simulink model "AirRefueling_Platform"  (R2022a)
settings: Solver=ode4  StartTime=0.0  StopTime=inf  FixedStep=0.01  RelTol=1e-5  AbsTol=1e-4  EnableMultiTasking=on
InitFcn:
  | F16_Init
values from neighbouring files (symbols this model uses):
  airSpeed = 393.72    [F16_Init.m]
  altitude = 9843    [F16_Init.m]
  d_f_rc = [3.75;0;-1.75]    [F16_Init.m]
  d_pr_cam = d_pr_rc - d_cam_rc    [F16_Init.m]
  d_pr_rc = [7.6;0.50;-2.44]    [F16_Init.m]
  p0_rc = [-250;-119;0]    [F16_Init.m]
  visual_err = [0.07;0.04;-1.21]    [F16_Init.m]
undefined symbols (not defined in the file or in its folder): Cdr_, dtheta10, dtheta20, F, height, k_reel, kd, l0, l1, l_density, Light, m0, Mdr, MIL, N, Rdr, Rl, STD, T_reel_initial, theta10, theta20, vt0
libraries: etargetslib x10, dspnetwork x10, simulink x2, aerolibconvert2 x2, aerolibwind2 x2, aerolibatmos2 x1, aerolibanimutils x1, slrealtimeiplib x1
(part 2 of 2)

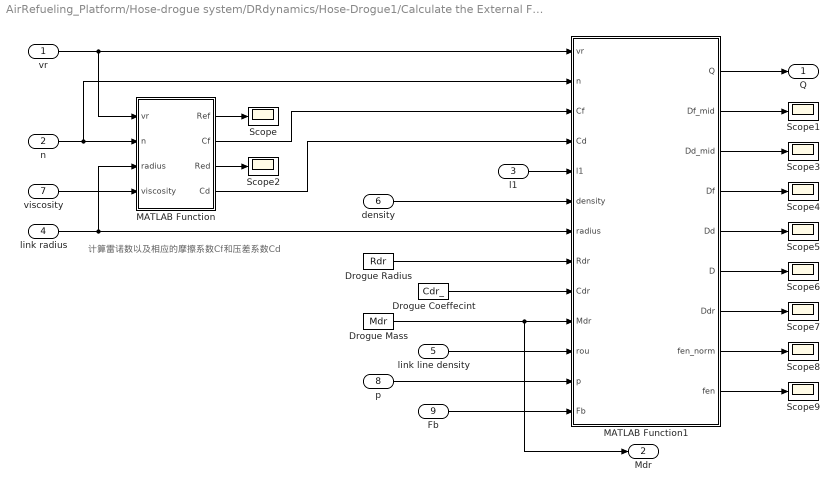
== system AirRefueling_Platform/Hose-drogue system/DRdynamics/Hose-Drogue1/Calculate the External Force of the Links ==
  note: 计算雷诺数以及相应的摩擦系数Cf和压差系数Cd
  vr : Inport
  n : Inport  Port=2
  l1 : Inport  Port=3
  link radius : Inport  Port=4
  link line density : Inport  Port=5
  density : Inport  Port=6
  viscosity : Inport  Port=7
  p : Inport  Port=8
  Fb : Inport  Port=9
  Drogue Coeffecint : Constant  Value=Cdr_
  Drogue Mass : Constant  Value=Mdr
  Drogue Radius : Constant  Value=Rdr
  MATLAB Function : MATLAB Function  TreatAsAtomicUnit=on
  MATLAB Function1 : MATLAB Function  TreatAsAtomicUnit=on
  Scope{,1..9} (10 alike) : Scope
  Q : Outport
  Mdr : Outport  Port=2
  wires:
  MATLAB Function/1(Ref) -> Scope/1
  MATLAB Function/3(Red) -> Scope2/1
  MATLAB Function1/1(Q) -> Q/1
  vr/1 -> MATLAB Function/1(vr), MATLAB Function1/1(vr)
  n/1 -> MATLAB Function1/2(n), MATLAB Function/2(n)
  link radius/1 -> MATLAB Function/3(radius), MATLAB Function1/7(radius)
  viscosity/1 -> MATLAB Function/4(viscosity)
  density/1 -> MATLAB Function1/6(density)
  Drogue Radius/1 -> MATLAB Function1/8(Rdr)
  Drogue Coeffecint/1 -> MATLAB Function1/9(Cdr)
  Drogue Mass/1 -> Mdr/1, MATLAB Function1/10(Mdr)
  link line density/1 -> MATLAB Function1/11(rou)
  MATLAB Function1/2(Df_mid) -> Scope1/1
  MATLAB Function1/3(Dd_mid) -> Scope3/1
  MATLAB Function1/4(Df) -> Scope4/1
  MATLAB Function1/5(Dd) -> Scope5/1
  MATLAB Function1/6(D) -> Scope6/1
  MATLAB Function1/7(Ddr) -> Scope7/1
  MATLAB Function/2(Cf) -> MATLAB Function1/3(Cf)
  MATLAB Function/4(Cd) -> MATLAB Function1/4(Cd)
  p/1 -> MATLAB Function1/12(p)
  l1/1 -> MATLAB Function1/5(l1)
  Fb/1 -> MATLAB Function1/13(Fb)
  MATLAB Function1/8(fen_norm) -> Scope8/1
  MATLAB Function1/9(fen) -> Scope9/1

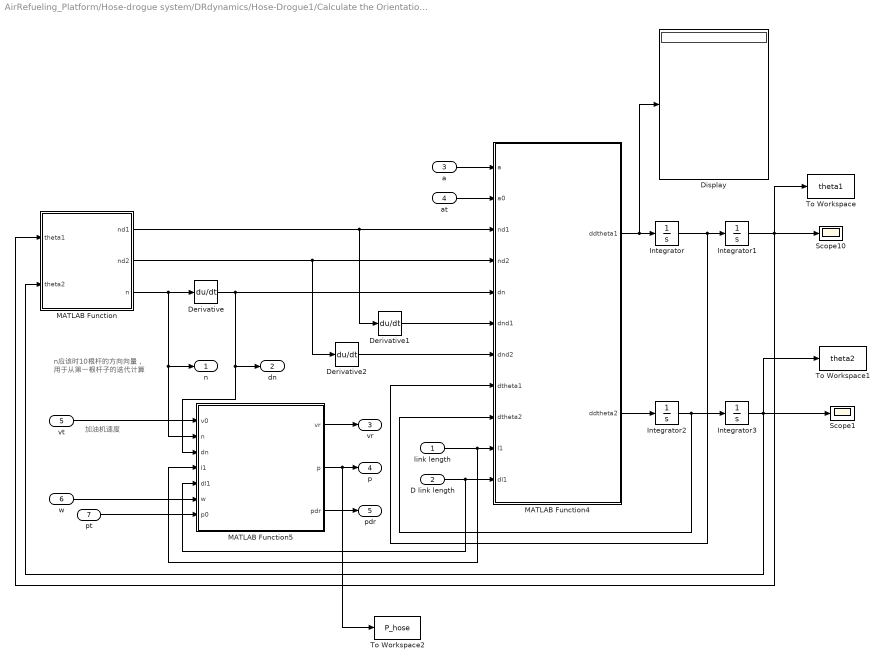
== system AirRefueling_Platform/Hose-drogue system/DRdynamics/Hose-Drogue1/Calculate the Orientation of the Links1 ==
  note: n应该时10根杆的方向向量，
      | 用于从第一根杆子的迭代计算
  note: 加油机速度
  link length : Inport
  D link length : Inport  Port=2
  a : Inport  Port=3
  at : Inport  Port=4
  vt : Inport  Port=5
  w : Inport  Port=6
  pt : Inport  Port=7
  Derivative : Derivative
  Derivative1 : Derivative
  Derivative2 : Derivative
  Display : Display
  Integrator : Integrator  InitialCondition=dtheta10
  Integrator1 : Integrator  InitialCondition=theta10
  Integrator2 : Integrator  InitialCondition=dtheta20
  Integrator3 : Integrator  InitialCondition=theta20
  MATLAB Function : MATLAB Function  TreatAsAtomicUnit=on
  MATLAB Function4 : MATLAB Function  TreatAsAtomicUnit=on
  MATLAB Function5 : MATLAB Function  TreatAsAtomicUnit=on
  Scope1 : Scope
  Scope10 : Scope
  To Workspace : ToWorkspace  VariableName=theta1  SampleTime=-1
      settings: Save2DSignal=2-D array (concatenate along first dimension)
  To Workspace1 : ToWorkspace  VariableName=theta2  SampleTime=-1
      settings: Save2DSignal=2-D array (concatenate along first dimension)
  To Workspace2 : ToWorkspace  VariableName=P_hose  SampleTime=-1
  n : Outport
  dn : Outport  Port=2
  vr : Outport  Port=3
  p : Outport  Port=4
  pdr : Outport  Port=5
  wires:
  Integrator1/1 -> To Workspace/1, MATLAB Function/1(theta1), Scope10/1
  Integrator3/1 -> To Workspace1/1, MATLAB Function/2(theta2), Scope1/1
  MATLAB Function/3(n) -> MATLAB Function5/2(n), n/1, Derivative/1
  Integrator/1 -> MATLAB Function4/8(dtheta1), Integrator1/1
  Integrator2/1 -> MATLAB Function4/9(dtheta2), Integrator3/1
  Derivative1/1 -> MATLAB Function4/6(dnd1)
  Derivative2/1 -> MATLAB Function4/7(dnd2)
  MATLAB Function4/2(ddtheta2) -> Integrator2/1
  link length/1 -> MATLAB Function4/10(l1), MATLAB Function5/4(l1)
  D link length/1 -> MATLAB Function5/5(dl1), MATLAB Function4/11(dl1)
  a/1 -> MATLAB Function4/1(a)
  at/1 -> MATLAB Function4/2(a0)
  vt/1 -> MATLAB Function5/1(v0)
  w/1 -> MATLAB Function5/6(w)
  MATLAB Function5/1(vr) -> vr/1
  pt/1 -> MATLAB Function5/7(p0)
  MATLAB Function/1(nd1) -> Derivative1/1, MATLAB Function4/3(nd1)
  MATLAB Function/2(nd2) -> Derivative2/1, MATLAB Function4/4(nd2)
  Derivative/1 -> MATLAB Function5/3(dn), dn/1, MATLAB Function4/5(dn)
  MATLAB Function5/3(pdr) -> pdr/1
  MATLAB Function5/2(p) -> To Workspace2/1, p/1
  MATLAB Function4/1(ddtheta1) -> Display/1, Integrator/1

== matlab function AirRefueling_Platform/SimToUE ==
  data: y output; PosRc input; PosTb1 input; Pos_dr2tx output
function [y,Pos_dr2tx] = SimToVR(PosRc,PosTb1)
%#codegen

%%函数名：SimToVR
%%用途  ：将软管锥套坐标输出转换为VR输入
%%输入  ：PosPr - 受油机坐标， PlsTb - 软管坐标数据
%%输出  ：VrPos - 软管和受油机VR位置，VrAngle - 旋转角度输出
%%作者  ：戴训华
%%时间  ：2014/3/19

Pos_rc2tx = PosRc(4:6);
% add PosPr1(4:6)存储的是受油机的姿态  模型中在输出姿态[phi, theta, psai]后加上了trim_state1=[0;0.1156,0],这里又给减掉了
% 无人机先绕机体系 z 轴旋转 ψ \psiψ，再绕机体系 y 轴旋转 θ \thetaθ，最后绕机体系 x 轴旋转 ϕ \phiϕ，[yaw,pitch,roll]
% AttitudeRecei = [PosPr1(4);-PosPr1(6);PosPr1(5)-0.115609];
AttitudeRecei = [0;0.1156;0];
PosTb = PosTb1(1:60);

% 这个不用 用的是通过最后一根杆子生成锥套的方法
PosDr = PosTb1(61:63);

% 这里是20根软管+1个锥套+1个受油机 
VrAngle = zeros(22*3,1);
VrPos = zeros(22*3,1);

% 对于发送模型的视觉修正  全部在这里
% 由于这里只管发送 所以必须让前面模型在计算时也考虑这些修正，这样才能把各种计算都对上
hose_delta_pos = [0;0;0];                      % 视觉对齐 让软管都上升1m
drogue_delta_pos =[0;0;.04];                   % 调整锥套的位置 让它和最后一根软管对上 和软管一样先调整1m，再微调 其实就是 hose_delta_pos + [0.85;0;-0.15]
drogue_delta_angle = [0;0;0];                  % 调整锥套的角度 让它和最后一根软管的角度切合 rpy，pitch向上是正向下是负 [0;-8/180*pi;pi] 
drogue_visual_pos = [-0.05;0;1.1];             % 这里要将锥套的位置反馈给前面做计算，要将锥套的视觉位置dr2tx+drogue_visual_pos=实际的锥套位置  
                                               % 方法是通过视觉识别得到的dr2cam(z)+cam2rc(z)+dr2tx(z)=rc2tx(z).这里dr2cam是准确的，只有dr2tx可变，所以修正到这里

% add
scale = 1;
for j = 1:21                        %前20为软管坐标数据，后1为软管平滑过渡处理
    if j == 1
        pX = [0, 0, 0]';            %软管起点
        pY = PosTb(3*j-2:3*j);      %软杆终点
                                    % 不用平滑的 直接用锥套的真实位置
    elseif j == 21                  %多加一段杆，做过渡
        pX = PosTb(3*j-5:3*j-3);
        pY = [PosTb(3*j-5)-0.7163*cos(8/180*pi),PosTb(3*j-4),PosTb(3*j-3)+0.7163*sin(8/180*pi)]';
    else
        pX = PosTb(3*j-5:3*j-3);
        pY = PosTb(3*j-2:3*j); 
    end
    
    pZ = (pX + pY)/2;                   %中点坐标

    %到VR中比例的缩放
    pZ = pZ * scale;
    
    vAxis = [0,0,-1]';                  %水平轴
    vTb = pY - pX;                      %杆的方向
    
    axis1 = null([vAxis';vTb']);        %获取垂直向量
    vRot = axis1(:,1)';                 %得到旋转轴
    
    if vRot(2) < 0
        vRot = -vRot;
    end
 
    yaw_xoz = asin(vTb(2) / sqrt(vTb(1)*vTb(1) + vTb(2)*vTb(2)+ vTb(3)*vTb(3)));
    pitch_z = pi - atan(vTb(3) / vTb(1));
%     pitch_z = atan(vTb(3) / vTb(1));
    roll = 0;   % 圆柱形hose，不用计算roll   
    VrAngle(3*j-2:3*j) = [yaw_xoz, pitch_z, roll];
    % 视觉对齐 让软管都上升hose_delta_posm
    VrPos(3*j-2:3*j) = [pZ(1);pZ(2);pZ(3)] + hose_delta_pos;
end
% add 发送的是受油机的位置
VrAngle(64:66)=[AttitudeRecei(1);AttitudeRecei(2);AttitudeRecei(3)];

pZ = Pos_rc2tx;
pZ = pZ * scale;
VrPos(3*22-2:3*22) = [pZ(1),pZ(2),pZ(3)]';


tmp1 = VrPos(1:60,:);                               % 软管位置
tmp2 = VrPos(61:63,:) + drogue_delta_pos;           % 锥套位置
tmp3 = VrPos(64:66,:) ;                             % 受油机位置 
tmp4 = VrAngle(1:60,:);                             % 软管角度
tmp5 = tmp4(58:60) + drogue_delta_angle;            % 锥套角度 使用的是最后一根软管的角度
tmp6 = VrAngle(64:66,:);                            % 受油机角度

tmp=[tmp1;tmp4;tmp2;tmp5;tmp3;tmp6];
y = tmp;

% 发送反馈给前面的锥套位置由于视觉上有差异，所以需要修正 但是实际上发送的是tmp2，并没有发送调整过的值 
Pos_dr2tx=tmp2+drogue_visual_pos;

== matlab function AirRefueling_Platform/Tanker system/   ==
  data: u input; y output
function y = WindTurFromTank(u)
%#codegen

y = TankerVortexWindField(u);

== matlab function AirRefueling_Platform/Hose-drogue system/DRdynamics/Hose-Drogue1/Calculate the Acceleration of the Links1/MATLAB Function2 ==
  data: t0 output size=1; T input; q input; t output
function [t0,t] = fcn(T,q)
% 由于编译报错所以用下面两行来替换第三行。
t = zeros(10,1);
t = inv(T)*q;
% t = T\q;
t0 = t(1);

== matlab function AirRefueling_Platform/Hose-drogue system/DRdynamics/Hose-Drogue1/Calculate the Acceleration of the Links1/MATLAB Function3 ==
  data: t input; Q input; n input; m1 input; Mdr input; a output; N parameter; m0 parameter
function a = fcn(t,Q,n,m1,Mdr, N,m0)
a = zeros(3,N);
a(:,1) = (t(1)*n(:,1) - t(2)*n(:,2) + Q(:,1))/m1;
for i = 2:N-1
    a(:,i) = (t(i)*n(:,i) - t(i+1)*n(:,i+1) + Q(:,i))/m0;
end
a(:,N) = (t(N)*n(:,N) + Q(:,N))/(m0/2 + Mdr);                %注意最后一个节点的质量！！

== matlab function AirRefueling_Platform/Hose-drogue system/DRdynamics/Hose-Drogue1/Calculate the Acceleration of the Links1/MATLAB Function4 ==
  data: n input; dn input; q output; Q input; m1 input; l1 input; ddl1 input; a0 input; N parameter; l0 parameter; m0 parameter
function q = fcn(n,dn,Q,m1,l1,ddl1,a0, N,l0,m0)

% n = 连杆的方向向量，想上为正 向量3*N
% Q = 连杆所受的合外力 向量3*N
% m = 连杆质量 向量1*N
% l = 连杆长度 向量1*N
% dl = 连杆长度的一阶导数 向量1*N
% ddl = 连杆长度的二阶导数 向量1*N
% a0 = 连接点的加速度 向量3*1

%%%%求张力t%%%%%%%%%%%%%%%%%%%%%%%%%%%%%%%%%%%%%%%%%%%%%%%%%%%%%%
q = zeros(N,1);
q(1,1) = m1*l1*dn(:,1)'*dn(:,1) - Q(:,1)'*n(:,1) + m1*a0'*n(:,1) - m1*ddl1;
q(2,1) = l0*dn(:,2)'*dn(:,2) + (1/m1*Q(:,1) - 1/m0*Q(:,2))'*n(:,2); % 可参考有关变长度连杆的《推导》
for i = 3:N
    q(i,1) = l0*dn(:,i)'*dn(:,i) + (1/m0*Q(:,i-1) - 1/m0*Q(:,i))'*n(:,i);
end

== matlab function AirRefueling_Platform/Hose-drogue system/Collision Detection/MATLAB Function1 ==
  settings: updateMethod=DISCRETE
  data: Pos_pr input; F output; V_pr input; Pos_dr input; V_dr input; Mdr input; visual_err input
function F = fcn(Pos_pr,V_pr,Pos_dr,V_dr,Mdr,visual_err)
% 在x方向，椎管刚接触到锥套的时候，两者差是0.2m，完全进入时两者差是0.8
% 在z方向，椎管在锥套最下沿的时候，两者差是0.21m，在正中间的时候是0.12m 感觉这个不准
% error =z^2+y^2-x^2; 
% error<0 代表在圆锥里面
% 当x进入一定范围之内时，才能计算误差
% 当前位置减去定点的位置 相当于把定点放在了原点 x^2 = y^2 + z^2 （x<0）
% 分成xyz三个方向进行误差计算 
% x的范围[-0.2,0.45]  yz的范围相同,就是x一定时，半径时y=z=x对应的圆形的范围[-y,y]
% 给定了x之后 要判断两个 第一个是在这个圆形范围内，第二个是距离圆心的距
F = zeros(3,1);
% modify = [0.66;-0.1;0.645]*0+[0.7;-0.1;0.8]*0;
modify = visual_err;
% 是锥套位置-椎管位置 初始值是大于0的
x = Pos_dr(1) - Pos_pr(1)+ modify(1);
y = Pos_dr(2) - Pos_pr(2)+ modify(2);
% 椎管的z坐标要反一下 
z = Pos_dr(3) - Pos_pr(3)+ modify(3);
Vel_relative = V_pr - V_dr;

error =z^2+y^2-x^2; 
Kp_p = 100;
Kp_v = 50; 
persistent f;     
if(isempty(f))
    f=[0;0;0];
end
if x<0.05
%     F(1)= 1000 * Mdr * (-x) + 500 * Mdr * (Vel_relative(1));
%     % y方向的
%     F(2)= 1000 * Mdr * (-y) + 500 * Mdr * (Vel_relative(2));
%     % z方向的
%     F(3)= 1500 * Mdr * (-z) + 500 * Mdr * (Vel_relative(3));
    if x>-0.05
    F(1)= 100 * Mdr * (-x) + 1 * Mdr * (Vel_relative(1));
    % y方向的
    F(2)= 20 * Mdr * (-y) + 2 * Mdr * (Vel_relative(2));
    % z方向的
    F(3)= 20 * Mdr * (-z) + 2 * Mdr * (Vel_relative(3));
    f = F;
    else
        F=f;
    end
end
% F = zeros(3,1);

== matlab function AirRefueling_Platform/Hose-drogue system/MATLAB Function ==
  data: P_dr input; P_link10 input; P_hose_dr output
function P_hose_dr = fcn(P_dr,P_link10)
% P_link20=zeros(3,20);
% P_link20(:,1) = P_link10(:,1)/2;
% P_link20(:,2) = P_link10(:,1);
% P_link20(:,3) = (P_link10(:,2)+P_link10(:,1))/2;
% P_link20(:,4) = P_link10(:,2);
% P_link20(:,5) = (P_link10(:,3)+P_link10(:,2))/2;
% P_link20(:,6) = P_link10(:,3);
% P_link20(:,7) = (P_link10(:,4)+P_link10(:,3))/2;
% P_link20(:,8) = P_link10(:,4);
% P_link20(:,9) = (P_link10(:,5)+P_link10(:,4))/2;
% P_link20(:,10) = P_link10(:,5);
% P_link20(:,11) = (P_link10(:,6)+P_link10(:,5))/2;
% P_link20(:,12) = P_link10(:,6);
% P_link20(:,13) = (P_link10(:,7)+P_link10(:,6))/2;
% P_link20(:,14) = P_link10(:,7);
% P_link20(:,15) = (P_link10(:,8)+P_link10(:,7))/2;
% P_link20(:,16) = P_link10(:,8);
% P_link20(:,17) = (P_link10(:,9)+P_link10(:,8))/2;
% P_link20(:,18) = P_link10(:,9);
% P_link20(:,19) = (P_link10(:,10)+P_link10(:,9))/2;
% P_link20(:,20) = P_link10(:,10);
% %P_link20(:,20) = P_dr;
% P_link20_V60 = reshape(P_link20,60,1);


%% 

x = P_link10(1,:);
y = P_link10(2,:);
z = P_link10(3,:);
n=length(x)-1;% B样条曲线有n+1个控制点
k=4;% 三次B样条，因此阶数=次数+1

% 用于储存生成的点
X=[];
Y=[];
Z=[];

Nik_u=zeros(1,n+1);% 用于储存基函数
nodevector=U_quasi_uniform(n,k);% 生成节点向量

for u=0:0.01:1-0.01% 循环次数决定组成B样条曲线点的总数量
    for j=1:n+1% 生成Bi,3这一系列基函数
        Nik_u(j)=BaseFunction(j,k,u,nodevector);
    end
    % 由于B样条曲线具有局部支撑性，因此只有u周围一定区间会参与到计算
    X=[X,x*Nik_u'];
    Y=[Y,y*Nik_u'];
    Z=[Z,z*Nik_u'];
end
% 根据三次B样条插值的结果得到20根管子的位置
P_link20=zeros(3,20);
index = 1;
for i=1:length(X)/20:100
    P_link20(:,index)=[X(i),Y(i),Z(i)];
    index = index+1;
end

P_link20_V60 = reshape(P_link20,60,1);
% 再将锥套的真实位置传过去 此时是63*1(20根管子+1个锥套)的向量 前面60个是软管 最后三个是锥套
P_hose_dr = [P_link20_V60;P_dr];

== matlab function AirRefueling_Platform/3D rendering engine/MATLAB Function ==
  settings: updateMethod=DISCRETE  sampleTime=0.01
  data: y output; t input
function y = fcn(t)
y = [-100 -119 -100];  % initial position
v1 = 15; % velocity
y(1) = y(1) + v1 * t;
end

== matlab function AirRefueling_Platform/Hose-drogue system/DRdynamics/Hose-Drogue1/Calculate the External Force of the Links/MATLAB Function ==
  data: vr input; n input; Ref output; radius input; viscosity input; Cf output; Red output; Cd output; N parameter
function [Ref, Cf, Red, Cd] = C(vr,n,radius,viscosity, N)
% 计算雷诺数以及相应的摩擦系数Cf和压差系数Cd

% 单杆的速度、方向等用3*1的列向量表示
% vr = 连杆相对风速度 向量3*N
% n = 连杆的方向向量，想上为正 向量3*N
% viscosity  = 动粘度系数
% radius = 连杆半径

%——计算雷诺数———————————————————————————
cosa = zeros(1,N);
sina = zeros(1,N);
Ref = zeros(1,N);
Red = zeros(1,N);
for i = 1:N
    if norm(vr(:,i)) ~= 0
        cosa(i) = vr(:,i)'*n(:,i)/norm(vr(:,i));
        sina(i) = sqrt(1-cosa(i)^2);
        if sina(i) ~= 0
            Ref(i) = (pi*radius/viscosity)*norm(vr(:,i))/sina(i);
        else
            Ref(i) = 10^11;
        end
        Red(i) = norm(vr(:,i))*2*radius/viscosity;
    end
end

%——计算气动系数——————————————————————————
Cf = zeros(1,N);
Cd = zeros(1,N);
for i = 1:N
    %%%%Cf表%%%%%%%%%%%%%%%%%%%%%%%%
    if Ref(i)<=10^-2
        Cf(i) = 0;    %注意这里有改动
    elseif Ref(i)>10^-2 && Ref(i)<=10^4
        Cf(i) = 4.6409*Ref(i)^-0.6667;
    elseif Ref(i)>10^4 && Ref(i)<=10^10
        Cf(i) = 0.0464*Ref(i)^-0.1667;
    elseif Ref(i)>10^10
        Cf(i) = 0.001;
    end
    %%%%Cd表%%%%%%%%%%%%%%%%%%%%%%%%%
    if Red(i)<=10^-2
        Cd(i) = 0;   %注意这里有改动
    elseif Red(i)>10^-2 && Red(i)<=1
        Cd(i) = 10*Red(i)^-0.801;
    elseif Red(i)>1 && Red(i)<=180
        Cd(i) = 10*Red(i)^-0.4083;
    elseif Red(i)>180 && Red(i)<=4*10^5
        Cd(i) = 1.2;
    elseif Red(i)>4*10^5 && Red(i)<=4*10^6
        Cd(i) = 0.002128*Red(i)^0.3522;
    elseif Red(i)>4*10^6
        Cd(i) = 0.45;
    end
end

== matlab function AirRefueling_Platform/Hose-drogue system/DRdynamics/Hose-Drogue1/Calculate the External Force of the Links/MATLAB Function1 ==
  data: vr input; Q output; n input; Cf input; Cd input; l1 input; density input; radius input; Rdr input; Cdr input; Mdr input; rou input; p input; Fb input; Df_mid output; Dd_mid output; Df output; Dd output; D output; Ddr output; N parameter; l0 parameter; fen_norm output; fen output
function [Q, Df_mid, Dd_mid, Df, Dd, D, Ddr, fen_norm, fen] = ExternalForce(vr,n,Cf,Cd,l1,density,radius,Rdr,Cdr,Mdr,rou,p,Fb, N,l0)

% 计算每根连杆的合外力

% 单杆的速度、方向等用3*1的列向量表示
% l = 每根连杆的长度，注意这里要做成变长的 向量
% vr = 连杆相对风速度 向量3*N
% n = 连杆的方向向量，想上为正 向量3*N
% viscosity  = 大气动粘度系数
% density = 大气密度
% radius = 连杆半径
% r_dr = 锥套伞冠半径
% rou = 连杆的线密度

% Cdr = 锥套的阻力系数
% Rdr = 锥套伞冠半径
% Mdr = 锥套质量

%——求气动力————————————————————————————
Df_mid = zeros(1,N);
Dd_mid = zeros(1,N);
Df = zeros(3,N);
Dd = zeros(3,N);
D = zeros(3,N);
vn = zeros(3,N);
for i = 1:N
    if i == 1
        Df_mid(i) = density*pi*radius*l1*Cf(i)*(vr(:,i)'*n(:,i))^2;
    else
        Df_mid(i) = density*pi*radius*l0*Cf(i)*(vr(:,i)'*n(:,i))^2;
    end
    if vr(:,i)'*n(:,i)>0   % 这里可能有符号问题，万一之后还是出现杂乱的情况，要注意这里
        Df(:,i) = Df_mid(i)*n(:,i);
    else
        Df(:,i) = - Df_mid(i)*n(:,i);
    end
    % 当杆的方向迎着风的时候，摩擦阻力延杆反向
    % 当杆的方向顺着风的时候，摩擦阻力延杆正向
    
    vn(:,i) = vr(:,i)-(vr(:,i)'*n(:,i))*n(:,i); 
    if i == 1
        if norm(vn(:,i)) ~= 0
            Dd_mid(i) = density*radius*l1*Cd(i)*norm(vn(:,i))^2;
            Dd(:,i) = - Dd_mid(i)*vn(:,i)/norm(vn(:,i));
        else
            Dd(:,i) = [0;0;0];
        end
    else
        if norm(vn(:,i)) ~= 0
            Dd_mid(i) = density*radius*l0*Cd(i)*norm(vn(:,i))^2;
            Dd(:,i) = - Dd_mid(i)*vn(:,i)/norm(vn(:,i));
        else
            Dd(:,i) = [0;0;0];
        end
    end
    % 无论连杆与相对速度的角度关系如何，压差阻力总是顺着风的方向的
        
    D(:,i) = Df(:,i) + Dd(:,i);
end

if vr(:,N)'*vr(:,N) ~= 0
    Ddr = - 1/2*density*vr(:,N)'*vr(:,N)*(pi*Rdr^2)*(Cdr)* vr(:,N)/norm(vr(:,N));
else
    Ddr = [0;0;0];
end
%%%%%%%%%%%%%%%%%%%%%%%%%%%%%%%%%%%%%%%%%%%%%%%%%%%%%%%%%%%%%%%%

% %%%%计算恢复力%%%%%%%%%%%%%%%%%%%%%%
do = 1; % 连杆外径
di = 0.84; % 连杆内径
E = 589.67; % 弹性系数 数量级可能有问题
K = E*pi/8*(do^4 - di^4);
fen_norm = zeros(1,N);
fen = zeros(3,N);
for i = 2:N-1
    n0mid = (p(:,i-1) - p(:,i+1))/norm(p(:,i-1) - p(:,i+1));
    if abs(norm(n(:,i-1)'*n(:,i))-1) ~= 0;
        gama1 = n(:,i-1)'*n0mid;
        gama2 = n(:,i)'*n0mid;
        if norm(gama1) >= 1
            gama1 = gama1/abs(gama1);
        end
        if norm(gama2) >= 1
            gama2 = gama2/abs(gama2);
        end
            
        fen_norm(i) = K*(acos(gama1) + acos(gama2))/norm(p(:,i-1) - p(:,i+1))^2;
        fen(:,i) = fen_norm(i)*((n(:,i)'*n0mid*n0mid - n(:,i))*1e3)/norm((n(:,i)'*n0mid*n0mid - n(:,i))*1e3);
    end
end
%%%%%%%%%%%%%%%%%%%%%%%%%%%%%%%%%%%%%%

% %%%%计算合外力%%%%%%%%%%%%%%%%%%%%%%?
% Q = zeros(3,N);
% for i = 1:N-1
%     Q(:,i) = [0;0;m*g] + 1/2*(D(:,i)+D(:,i+1));
% end
% Q(:,N) = [0;0;(m+Mdr)*g] + 1/2*D(:,N) + Ddr;
Q = zeros(3,N);
Q(:,1) = [0;0;l1*rou*9.8] + 1/2*(D(:,1)+D(:,2)) + fen(:,1);
for i = 2:N-1
    Q(:,i) = [0;0;l0*rou*9.8] + 1/2*(D(:,i)+D(:,i+1)) + fen(:,i);
end
Q(:,N) = [0;0;(l0/2*rou + Mdr)*9.8] + 1/2*D(:,N) + Ddr + Fb;        %注意最后一个节点的质量
% 这里删掉了锥套的受力（Bow wave），后面再处理
% %%%%%%%%%%%%%%%%%%%%%%%%%%%%%%%%

== matlab function AirRefueling_Platform/Hose-drogue system/DRdynamics/Hose-Drogue1/Calculate the Orientation of the Links1/MATLAB Function ==
  data: nd1 output; nd2 output; theta1 input; n output; theta2 input; N parameter
function [nd1,nd2,n] = fcn(theta1,theta2, N)
% theta1,theta2 向量1*n
n = zeros(3,N);
nd1 = zeros(3,N);
nd2 = zeros(3,N);

for i = 1:N
    n(:,i) = [cos(theta1(i))*cos(theta2(i)); sin(theta2(i)); -sin(theta1(i))*cos(theta2(i))];
    nd1(:,i) = [-sin(theta1(i))*cos(theta2(i)); 0; -cos(theta1(i))*cos(theta2(i))];
    nd2(:,i) = [-cos(theta1(i))*sin(theta2(i)); cos(theta2(i)); sin(theta1(i))*sin(theta2(i))];
end

== matlab function AirRefueling_Platform/Hose-drogue system/DRdynamics/Hose-Drogue1/Calculate the Orientation of the Links1/MATLAB Function4 ==
  data: a input; a0 input; nd1 input; nd2 input; dn input; dnd1 input; dnd2 input; dtheta1 input; dtheta2 input; l1 input size=1; dl1 input; ddtheta1 output; ddtheta2 output; N parameter; l0 parameter
function [ddtheta1,ddtheta2] = fcn(a,a0,nd1,nd2,dn,dnd1,dnd2,dtheta1,dtheta2,l1,dl1, N, l0)
% theta1,theta2 向量N*1
% omiga,alpha是加油机坐标系的旋转角速度和叫加速度
% a是各节点的加速度
% a0为加油机加速度
% l,dl,ddl是连杆的长度及其一二阶导数

ddtheta1 = zeros(1,N);
ddtheta2 = zeros(1,N);

ddtheta1(1) = nd1(:,1)'*(-(a(:,1)-a0)-2*dl1*dn(:,1)-...
              l1*(dnd1(:,1)*dtheta1(1)+dnd2(:,1)*dtheta2(1)))...
              /(l1*norm(nd1(:,1)));
ddtheta2(1) = nd2(:,1)'*(-(a(:,1)-a0)-2*dl1*dn(:,1)-...
              l1*(dnd1(:,1)*dtheta1(1)+dnd2(:,1)*dtheta2(1)))...
              /(l1*norm(nd2(:,1)));
for i = 2:N
    ddtheta1(i) = nd1(:,i)'*(-(a(:,i)-a(:,i-1))-...
                  l0*(dnd1(:,i)*dtheta1(i)+dnd2(:,i)*dtheta2(i)))...
                  /(l0*norm(nd1(:,i)));
    ddtheta2(i) = nd2(:,i)'*(-(a(:,i)-a(:,i-1))-...
                  l0*(dnd1(:,i)*dtheta1(i)+dnd2(:,i)*dtheta2(i)))...
                  /(l0*norm(nd2(:,i)));
end

== matlab function AirRefueling_Platform/Hose-drogue system/DRdynamics/Hose-Drogue1/Calculate the Orientation of the Links1/MATLAB Function5 ==
  data: v0 input; n input; dn input; l1 input; dl1 input; w input; vr output; p0 input; p output; N parameter; l0 parameter; pdr output
function [vr,p,pdr] = fcn(v0,n,dn,l1,dl1,w,p0, N, l0)

% v0为加油机速度
% l,dl是连杆的长度及其一阶导数
% wt为合成风在每个节点的风速
% p0为预留，在计算相对地面的位置时用到

vr = zeros(3,N);
vr(:,1) = v0 - dl1*n(:,1) - l1*dn(:,1) ;
for i = 2:N
    vr(:,i) = vr(:,i-1) - l0*dn(:,i);
end
vr = vr - w;

p = zeros(3,N);
p(:,1) = [0;0;0] - l1*n(:,1);
for i = 2:N
    p(:,i) = p(:,i-1) - l0*n(:,i);
end
pdr = p(:,N) + [-0.3;0;0];
% pdr = p(:,N);

== matlab function AirRefueling_Platform/Hose-drogue system/DRdynamics/Hose-Drogue1/MATLAB Function3 ==
  data: n input; alpha output; N parameter
function alpha = fcn(n, N)
% 计算两杆之间的弯折角度，用来粗略的验证恢复力的效果
alpha = zeros(1,N);
for i = 2:N
    mid = n(:,i-1)'*n(:,i);
    if abs(mid) > 1
        mid = mid/abs(mid);
    end
    alpha(i) = acos(mid)/pi*180;
end

== matlab function AirRefueling_Platform/Visual process/VehicleDataParse ==
  data: Data input; CopterID output; Length input; Out output; checksum input; len input
function [CopterID,Out] = fcn(Data,Length,checksum,len)

% 设定静态变量，在数据校验失败时，保持上一时刻值
persistent DataOut;
if isempty(DataOut)
    DataOut=zeros(16,1);
end
persistent cpID;
if isempty(cpID)
    cpID=0;
end

% 如果包长不等于设定值，这个包丢弃，使用原来的值
if Length ~= len %如果包长度不匹配，校验不通过，那么使用上一时刻值
    Out=DataOut;
    CopterID=cpID;
    return;
end

CkSum = typecast(Data(1:4), 'int32');
if CkSum ~= checksum %如果校验码不匹配，校验不通过，那么使用上一时刻值
    Out=DataOut;
    CopterID=cpID;
    return;    
end

% 提取数据
CpIDTmp = typecast(Data(5:8), 'int32');
DataTmp = typecast(Data(9:136), 'double');
% DataTmp=zeros(16,1);
for i=1:16
    idx = (i-1)*8+9;
    DataTmp(i) = typecast(Data(idx:idx+7), 'double');
end



% 配置输出数据
CopterID = double(CpIDTmp);
Out = DataTmp;

% 记录上一时刻值
cpID=CopterID;
DataOut=Out;

== matlab function AirRefueling_Platform/Hose-drogue system/DRdynamics/Hose-Drogue1/Calculate the Acceleration of the Links1/MATLAB Function ==
  data: n input; m1 input; T output; m0 parameter; N parameter
function T = fcn(n,m1, m0,N)

% n = 连杆的方向向量，想上为正 向量3*N
% m = 连杆的质量 向量1*N

%%%%求张力t%%%%%%%%%%%%%%%%%%%%%%%%%%%%%%%%%%%%%%%%%%%%%%%%%%%%%%
T = zeros(N,N);

T(1,1) = 1;
T(1,2) = - n(:,1)'*n(:,2);
T(N,N-1) = -1/m0*n(:,N-1)'*n(:,N);
T(N,N) = 1/m0 + 1/m0;             %注意这里很重要！！

T(2,1) = -1/m1*n(:,1)'*n(:,2);
T(2,2) = 1/m1 + 1/m0;
T(2,3) = -1/m0*n(:,2)'*n(:,3);

for i = 3:N-1
    T(i,i-1) = -1/m0*n(:,i-1)'*n(:,i);
    T(i,i) = 1/m0 + 1/m0;
    T(i,i+1) = -1/m0*n(:,i)'*n(:,i+1);
end

== matlab function AirRefueling_Platform/Tanker system/  ==
  data: u input; y output

function y = WindTurFromTank(u)
%#codegen

%横纵向气流角速度等下计算长度
c_lat=4;
c_lon=4;

%两端参考点
u1 = u+[0 ,c_lat ,0]';
u2 = u+[0 ,-c_lat, 0]';

yy1 = TankerVortexWindField(u1);
yy2 = TankerVortexWindField(u2);

%计算x轴向滚转角速度
yp = (yy1(3) - yy2(3))/4/c_lat;

u3=u+[c_lon, 0,0]';
u4=u+[-c_lon ,0,0]';
yy3 = TankerVortexWindField(u3);
yy4 = TankerVortexWindField(u4);

%俯仰角速度计算
yq = -(yy3(3) - yy4(3))/4/c_lon;

%偏航角速度设为0
yr = 0;

%质心处风场计算
y_uvw = TankerVortexWindField(u);


%y = [y_uvw(1);y_uvw(2);y_uvw(3);-yp;-yq;-yr]*0.5;
y = [y_uvw(1);y_uvw(2);y_uvw(3);-yp;-yq;-yr];

== matlab function AirRefueling_Platform/Hose-drogue system/DRdynamics/HDU/MATLAB Function1 ==
  data: l1 input; l1initial input; dl1 input; flag1 output size=1; l1out output; dl1out output; ddl1 input; ddl1out output
function [flag1,l1out,dl1out,ddl1out] = fcn(l1,l1initial,dl1,ddl1)
% 如果第一根管子的长度比初始值大 或者 第一根管子的加速度>0 那么就是要控制了 flag从0变1开始积分
if (l1 > l1initial) || (l1 == l1initial && dl1 > 0)
    flag1 = 1;
    l1out = l1initial;
    dl1out = 0;
    ddl1out = 0;
else
    flag1 = 0;
    l1out = l1;
    dl1out = dl1;
    ddl1out = ddl1;
end

== matlab function AirRefueling_Platform/Hose-drogue system/Bow Wave Effect/Bow Wave Effect Function ==
  data: x input; Fx output; y input; z input; Fy output; Fz output
function [Fx,Fy,Fz] = F_rc2dr(x,y,z)
Cx1 = 91.6170;
Cx2 = 0.3220;
Cx3 = 3.8870;
Cx4 = 2.7359;
Cx5 = 2.4939;
Cx6 = 309.7709;
Cx7 = 0.3237;
Cx8 = 0.3851;
Cx9 = 1.1471;

Cy1 = 223.3210;
Cy2 = 0.2082;
Cy3 = 0.8102;
Cy4 = 0.6555;

Cz1 = 173.2021;
Cz2 = 0.2141;
Cz3 = 0.5697;
Cz4 = 0.7038;

if x > 5.6493
    Fx = 0;
elseif x > 3.0893
    Fx = Cx1*(1-Cx2*(x-Cx3)^2)*exp(-y^2/Cx4)*exp(z/Cx5);
else
    Fx = Cx1*(1-Cx2*(x-Cx3)^2)*exp(-y^2/Cx4)*exp(z/Cx5)...
       + Cx6*(1-Cx7*x)*exp(-y^2/Cx8)*exp(z/Cx9);
end

if x > 4.8031
    Fy = 0;
else
    Fy = Cy1*(1-Cy2*x)*(y*exp(-y^2/Cy3))*exp(z/Cy4);
end

if x > 4.6275
    Fz = 0;
else
    Fz = -Cz1*(1-Cz2*x)*exp(-y^2/Cz3)*exp(z/Cz4);
end

== matlab function AirRefueling_Platform/Hose-drogue system/Total Turbulence   ==
  data: u1 input; u input; y output
function y = Dr_wind2Frc(u1,u)
%#codegen

Ve=120;
rho = 0.98;
Q=0.5*rho*Ve^2;
S=0.38;
CD=0.81*0.8;

uu=u(1);
vv=u(2);
ww=u(3);

%beta = acos(sqrt(vv^2+ww^2)/abs(uu));
%theta = atan(ww/vv);

C_beta = 0.3979;

yx=rho*S*CD*Ve*uu;
yy=Q*S*C_beta*vv/Ve;
yz=Q*S*C_beta*ww/Ve;

% 这个y_v是有涡流+自然风所得到的速度换算成的位置偏移
y_v = [yx,yy,yz]';
y=[y_v;u1+y_v];

== matlab function AirRefueling_Platform/Hose-drogue system/DRdynamics/HDU/MATLAB Function2 ==
  data: l_1 input; T0 input; Tt output size=1; t input; dl input; l1 parameter; k_reel parameter; kd parameter
function Tt = fcn(l_1,T0,t,dl, l1,k_reel,kd)
Treel = T0*(l_1/l1)^k_reel;
Tt = t - Treel - kd*dl;

== matlab function AirRefueling_Platform/Visual process/MATLAB Function ==
  data: u input; y output; data input
function y= fcn(u, data)
y = u;
if int64(y(4)) == 0
    y(1:3) = data;
end
